simulink model "Pitch_Controller_Generated_SFunc_org"  (Simulink 10.0)
settings: Solver=FixedStepDiscrete  StartTime=0.0  StopTime=80  FixedStep=Ts_pitch_controller  MaxStep=0.01  RelTol=1e-6  EnableMultiTasking=on
PreLoadFcn:
  | Pitch_Controller_Data_Dictionary
undefined symbols (not defined in the file): Actuator_Lookup_angle, Actuator_Lookup_extension, DiscIntNeverNeededParam, P_VAR_alpha_max, P_VAR_alpha_min, P_VAR_Blade_Length, P_VAR_emergency_brake_pitch_angle, P_VAR_LUT_max_pitch_angle, P_VAR_park_pitch_angle, P_VAR_Rotor_nominal_rpm, PARAM_PCTRL_alpha_Igain, PARAM_PCTRL_alpha_Pgain, PARAM_PCTRL_Dgain, PARAM_PCTRL_Igain, PARAM_PCTRL_Pgain, radps2rpm
Description:
  | Copyright 2009-2017 The MathWorks, Inc. The MathWorks, Inc.
settings Model: Creator=raarenst  LastModifiedBy=annonymous
settings DataIOCC: ExternalInput=pitch_ctrl_inputs  SignalLoggingSaveFormat=ModelDataLogs  SaveOutput=off  SignalLogging=off  SaveTime=off  OutputSaveName=ValveCommandOL
settings OptimizationCC: DefaultParameterBehavior=Inlined  ExpressionDepthLimit=2147483647  ZeroExternalMemoryAtStartup=off  ZeroInternalMemoryAtStartup=off  NoFixptDivByZeroProtection=on  EfficientFloat2IntCast=on  LifeSpan=1  EfficientTunableParamExpr=on
settings DebuggingCC: SignalInfNanChecking=error  SolverPrmCheckMsg=warning  FcnCallInpInsideContextMsg=warning  UniqueDataStoreMsg=error  AllowSymbolicDim=off  StateNameClashWarn=warning
settings HardwareCC: ProdLargestAtomicInteger=Long  ProdLargestAtomicFloat=Double  ProdIntDivRoundTo=Zero  ProdEndianess=BigEndian  ProdHWDeviceType=Freescale->32-bit PowerPC
settings ModelReferenceCC: ModelReferenceNumInstancesAllowed=Single
settings RTWCC: Description=Real-Time Workshop Embedded Coder  SystemTargetFile=ert.tlc  TemplateMakefile=ert_default_tmf  GenerateReport=on  IncludeHyperlinkInReport=on  LaunchReport=on  CreateSILPILBlock=SIL  GenerateTraceInfo=on  GenerateTraceReport=on  GenerateTraceReportSl=on  GenerateTraceReportSf=on  GenerateTraceReportEml=on
settings CodeAppCC: IgnoreTestpoints=on  CustomSymbolStrType=$N$R$M  CustomSymbolStrModelFcn=$N  InternalIdentifier=Classic
settings ERTTargetCC: MultiwordLength=2048  GenerateSampleERTMain=on  SuppressErrorStatus=on  SupportAbsoluteTime=off  SupportNonFinite=off  SupportComplex=off  InlinedParameterPlacement=NonHierarchical  ERTCustomFileTemplate=example_file_process.tlc  ConvertIfToSwitch=off  SuppressUnreachableDefaultCases=off
settings ConfigComp: CovExternalEMLEnable=off  CovSFcnEnable=off

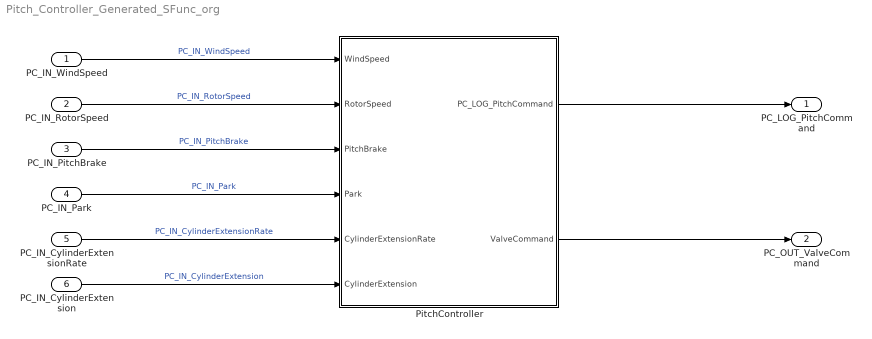
== system Pitch_Controller_Generated_SFunc_org ==
  PC_IN_WindSpeed : Inport  OutDataTypeStr=single
  PC_IN_RotorSpeed : Inport  Port=2  OutDataTypeStr=single
  PC_IN_PitchBrake : Inport  Port=3  OutDataTypeStr=boolean
  PC_IN_Park : Inport  Port=4  OutDataTypeStr=boolean
  PC_IN_CylinderExtensionRate : Inport  Port=5  OutDataTypeStr=single  PortDimensions=3
  PC_IN_CylinderExtension : Inport  Port=6  OutDataTypeStr=single  PortDimensions=3
  PitchController : Subsystem
  PC_LOG_PitchCommand : Outport  OutDataTypeStr=single
  PC_OUT_ValveCommand : Outport  Port=2  OutDataTypeStr=single
  wires:
  PitchController/2(ValveCommand) -> PC_OUT_ValveCommand/1
  PC_IN_WindSpeed/1 -> PitchController/1(WindSpeed)  "PC_IN_WindSpeed"
  PC_IN_RotorSpeed/1 -> PitchController/2(RotorSpeed)  "PC_IN_RotorSpeed"
  PC_IN_PitchBrake/1 -> PitchController/3(PitchBrake)  "PC_IN_PitchBrake"
  PC_IN_Park/1 -> PitchController/4(Park)  "PC_IN_Park"
  PC_IN_CylinderExtensionRate/1 -> PitchController/5(CylinderExtensionRate)  "PC_IN_CylinderExtensionRate"
  PC_IN_CylinderExtension/1 -> PitchController/6(CylinderExtension)  "PC_IN_CylinderExtension"
  PitchController/1(PC_LOG_PitchCommand) -> PC_LOG_PitchCommand/1

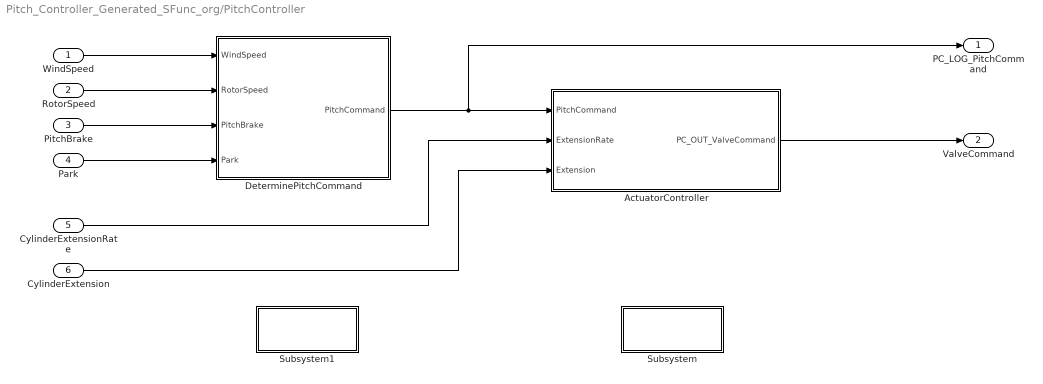
== system Pitch_Controller_Generated_SFunc_org/PitchController ==
  WindSpeed : Inport
  RotorSpeed : Inport  Port=2
  PitchBrake : Inport  Port=3
  Park : Inport  Port=4
  CylinderExtensionRate : Inport  Port=5
  CylinderExtension : Inport  Port=6
  ActuatorController : Subsystem
  DeterminePitchCommand : Subsystem
  Subsystem : Subsystem
      mask Display: disp('Inner loop')
  Subsystem1 : Subsystem
      mask Display: disp('Outer loop')
  PC_LOG_PitchCommand : Outport
  ValveCommand : Outport  Port=2
  wires:
  CylinderExtensionRate/1 -> ActuatorController/2(ExtensionRate)
  Park/1 -> DeterminePitchCommand/4(Park)
  PitchBrake/1 -> DeterminePitchCommand/3(PitchBrake)
  ActuatorController/1(PC_OUT_ValveCommand) -> ValveCommand/1
  RotorSpeed/1 -> DeterminePitchCommand/2(RotorSpeed)
  WindSpeed/1 -> DeterminePitchCommand/1(WindSpeed)
  CylinderExtension/1 -> ActuatorController/3(Extension)
  DeterminePitchCommand/1(PitchCommand) -> ActuatorController/1(PitchCommand), PC_LOG_PitchCommand/1

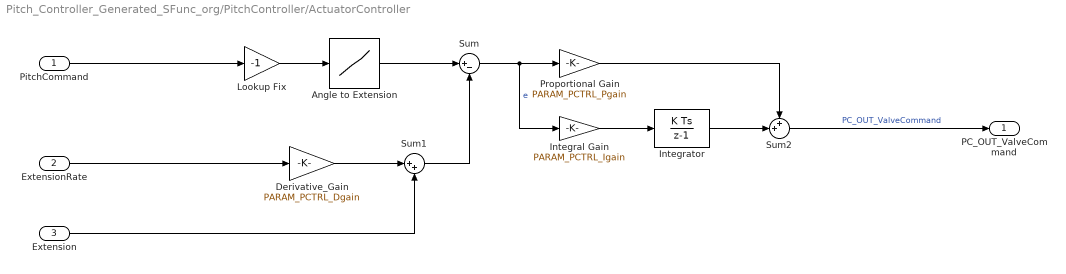
== system Pitch_Controller_Generated_SFunc_org/PitchController/ActuatorController ==
  PitchCommand : Inport
  ExtensionRate : Inport  Port=2
  Extension : Inport  Port=3
  Angle to Extension : Lookup  InputValues=Actuator_Lookup_angle  Table=Actuator_Lookup_extension
  Derivative_Gain : Gain  Gain=PARAM_PCTRL_Dgain
  Integral Gain : Gain  Gain=PARAM_PCTRL_Igain  SaturateOnIntegerOverflow=on  OutDataTypeStr=Inherit: Same as input  ParamDataTypeStr=Inherit: Same as input
  Integrator : DiscreteIntegrator  SampleTime=-1  ICPrevOutput=DiscIntNeverNeededParam  ICPrevScaledInput=DiscIntNeverNeededParam  mask(DiscretizedDiscreteIntegrator){}
      mask init:
      | %zoh
      settings: AttributesFormatString=Ts=%<SampleTime>\nIC_Mode=%<InitialConditionMode>
  Lookup Fix : Gain  Gain=-1
  Proportional Gain : Gain  Gain=PARAM_PCTRL_Pgain  SaturateOnIntegerOverflow=on  OutDataTypeStr=Inherit: Same as input  ParamDataTypeStr=Inherit: Same as input
  Sum : Sum  Inputs=|+-  InputSameDT=on
  Sum1 : Sum  Inputs=|++  InputSameDT=on
  Sum2 : Sum  Inputs=++|  SaturateOnIntegerOverflow=on  InputSameDT=on  OutDataTypeStr=Inherit: Same as first input
  PC_OUT_ValveCommand : Outport
  wires:
  Extension/1 -> Sum1/2
  Derivative_Gain/1 -> Sum1/1
  ExtensionRate/1 -> Derivative_Gain/1
  PitchCommand/1 -> Lookup Fix/1
  Angle to Extension/1 -> Sum/1
  Lookup Fix/1 -> Angle to Extension/1
  Sum1/1 -> Sum/2
  Integral Gain/1 -> Integrator/1
  Proportional Gain/1 -> Sum2/1
  Integrator/1 -> Sum2/2
  Sum2/1 -> PC_OUT_ValveCommand/1  "PC_OUT_ValveCommand"
  Sum/1 -> Proportional Gain/1, Integral Gain/1  "e"

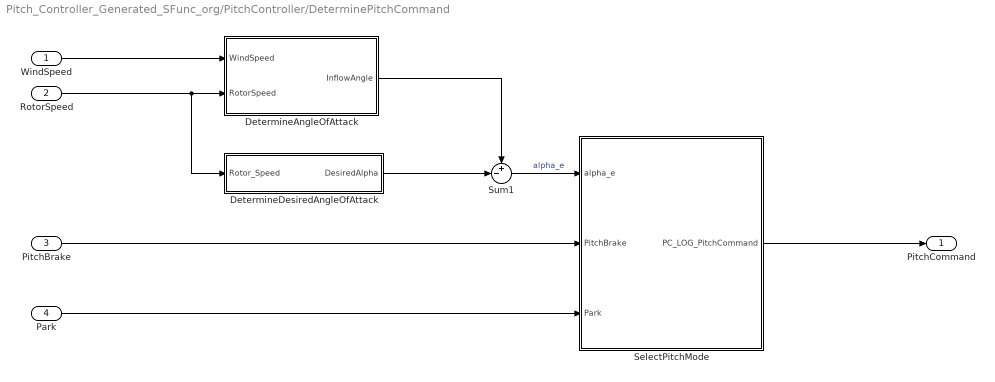
== system Pitch_Controller_Generated_SFunc_org/PitchController/DeterminePitchCommand ==
  WindSpeed : Inport
  RotorSpeed : Inport  Port=2
  PitchBrake : Inport  Port=3
  Park : Inport  Port=4
  DetermineAngleOfAttack : Subsystem
  DetermineDesiredAngleOfAttack : Subsystem
  SelectPitchMode : Subsystem
  Sum1 : Sum  Inputs=+-|  OutDataTypeStr=single  InputSameDT=on
  PitchCommand : Outport
  wires:
  Park/1 -> SelectPitchMode/3(Park)
  PitchBrake/1 -> SelectPitchMode/2(PitchBrake)
  DetermineDesiredAngleOfAttack/1(DesiredAlpha) -> Sum1/2
  DetermineAngleOfAttack/1(InflowAngle) -> Sum1/1
  RotorSpeed/1 -> DetermineAngleOfAttack/2(RotorSpeed), DetermineDesiredAngleOfAttack/1(Rotor_Speed)
  WindSpeed/1 -> DetermineAngleOfAttack/1(WindSpeed)
  SelectPitchMode/1(PC_LOG_PitchCommand) -> PitchCommand/1
  Sum1/1 -> SelectPitchMode/1(alpha_e)  "alpha_e"

== system Pitch_Controller_Generated_SFunc_org/PitchController/Subsystem ==

== system Pitch_Controller_Generated_SFunc_org/PitchController/Subsystem1 ==

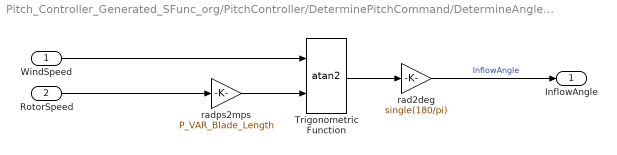
== system Pitch_Controller_Generated_SFunc_org/PitchController/DeterminePitchCommand/DetermineAngleOfAttack ==
  WindSpeed : Inport
  RotorSpeed : Inport  Port=2
  Trigonometric Function : Trigonometry  Operator=atan2
  rad2deg : Gain  Gain=single(180/pi)
  radps2mps : Gain  Gain=P_VAR_Blade_Length
  InflowAngle : Outport
  wires:
  radps2mps/1 -> Trigonometric Function/2
  Trigonometric Function/1 -> rad2deg/1
  WindSpeed/1 -> Trigonometric Function/1
  RotorSpeed/1 -> radps2mps/1
  rad2deg/1 -> InflowAngle/1  "InflowAngle"

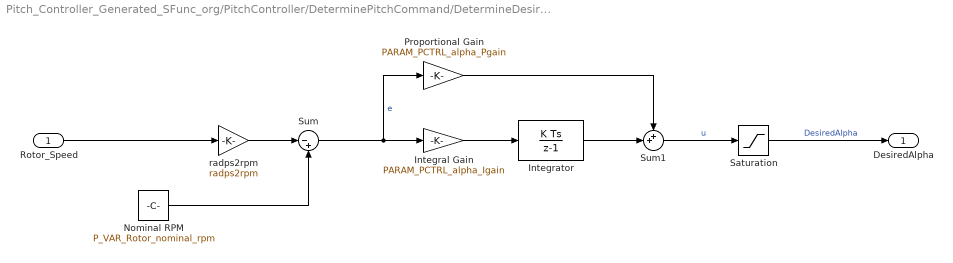
== system Pitch_Controller_Generated_SFunc_org/PitchController/DeterminePitchCommand/DetermineDesiredAngleOfAttack ==
  Rotor_Speed : Inport
  Integral Gain : Gain  Gain=PARAM_PCTRL_alpha_Igain  SaturateOnIntegerOverflow=on  OutDataTypeStr=Inherit: Same as input  ParamDataTypeStr=Inherit: Same as input
  Integrator : DiscreteIntegrator  SampleTime=-1  LimitOutput=on  UpperSaturationLimit=P_VAR_alpha_max  LowerSaturationLimit=P_VAR_alpha_min  ICPrevOutput=DiscIntNeverNeededParam  ICPrevScaledInput=DiscIntNeverNeededParam  mask(DiscretizedDiscreteIntegrator){}
      mask init:
      | %zoh
      settings: AttributesFormatString=Ts=%<SampleTime>\nIC_Mode=%<InitialConditionMode>
  Nominal RPM : Constant  Value=P_VAR_Rotor_nominal_rpm  OutDataTypeStr=single
  Proportional Gain : Gain  Gain=PARAM_PCTRL_alpha_Pgain  SaturateOnIntegerOverflow=on  OutDataTypeStr=Inherit: Same as input  ParamDataTypeStr=Inherit: Same as input
  Saturation : Saturate  UpperLimit=P_VAR_alpha_max  LowerLimit=-inf
      settings: AttributesFormatString=Upper=%<UpperLimit>\nLower=%<LowerLimit>
  Sum : Sum  Inputs=|-+  InputSameDT=on
  Sum1 : Sum  Inputs=++|  SaturateOnIntegerOverflow=on  InputSameDT=on  OutDataTypeStr=Inherit: Same as first input
  radps2rpm : Gain  Gain=radps2rpm
  DesiredAlpha : Outport
  wires:
  Nominal RPM/1 -> Sum/2
  radps2rpm/1 -> Sum/1
  Rotor_Speed/1 -> radps2rpm/1
  Saturation/1 -> DesiredAlpha/1  "DesiredAlpha"
  Sum1/1 -> Saturation/1  "u"
  Integral Gain/1 -> Integrator/1
  Proportional Gain/1 -> Sum1/1
  Integrator/1 -> Sum1/2
  Sum/1 -> Integral Gain/1, Proportional Gain/1  "e"

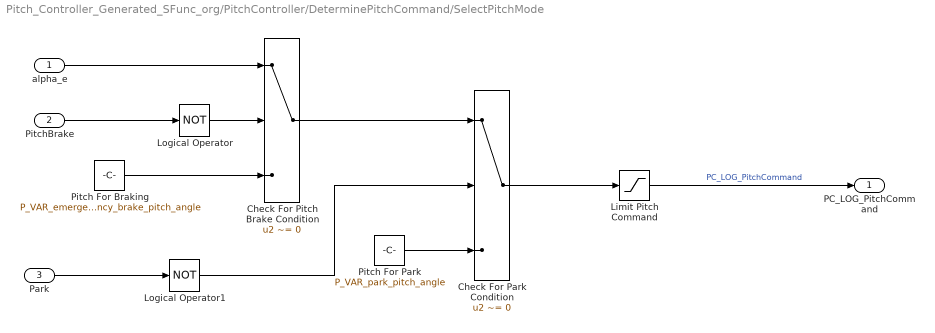
== system Pitch_Controller_Generated_SFunc_org/PitchController/DeterminePitchCommand/SelectPitchMode ==
  alpha_e : Inport
  PitchBrake : Inport  Port=2
  Park : Inport  Port=3
  Check For Park Condition : Switch  Criteria=u2 ~= 0  InputSameDT=on
      settings: AttributesFormatString=Criteria: %<Criteria>
  Check For Pitch Brake Condition : Switch  Criteria=u2 ~= 0  InputSameDT=on
      settings: AttributesFormatString=Criteria: %<Criteria>
  Limit Pitch Command : Saturate  UpperLimit=P_VAR_LUT_max_pitch_angle  LowerLimit=P_VAR_emergency_brake_pitch_angle
      settings: AttributesFormatString=Upper=%<UpperLimit>\nLower=%<LowerLimit>
  Logical Operator : Logic  Operator=NOT  AllPortsSameDT=off  OutDataTypeStr=boolean
  Logical Operator1 : Logic  Operator=NOT  AllPortsSameDT=off  OutDataTypeStr=boolean
  Pitch For Braking : Constant  Value=P_VAR_emergency_brake_pitch_angle  OutDataTypeStr=single
  Pitch For Park : Constant  Value=P_VAR_park_pitch_angle  OutDataTypeStr=single
  PC_LOG_PitchCommand : Outport
  wires:
  Check For Park Condition/1 -> Limit Pitch Command/1
  Logical Operator/1 -> Check For Pitch Brake Condition/2
  Pitch For Braking/1 -> Check For Pitch Brake Condition/3
  Logical Operator1/1 -> Check For Park Condition/2
  Pitch For Park/1 -> Check For Park Condition/3
  Check For Pitch Brake Condition/1 -> Check For Park Condition/1
  alpha_e/1 -> Check For Pitch Brake Condition/1
  PitchBrake/1 -> Logical Operator/1
  Limit Pitch Command/1 -> PC_LOG_PitchCommand/1  "PC_LOG_PitchCommand"
  Park/1 -> Logical Operator1/1
